simulink model "vipldws"  (R2017b)
settings: Solver=FixedStepDiscrete  StartTime=0.0  StopTime=inf  RelTol=1e-3  EnableMultiTasking=on
model workspace (MATLAB code in the model file):
  | % Image size
  | imgSize = [240 360];
  | 
  | % Number of rows and columns in the image region to process.
  | numRows = floor(imgSize(1)/2);
  | numCols = imgSize(2);
  | 
  | % To handle different video sizes other than [240 360], scaling the Hough
  | % transform rho values by the below factor is required.
  | factor = sqrt(sum(imgSize.^2)) / sqrt(sum([240 360].^2));
  | 
  | %% parameters for the second lane
  | %approximately 35:45 (0-based index: 414:424)
  | startIdxRho_R = floor(factor * 414);
  | NumRhos_R = floor(factor * 11);
  | 
  | %approximately -90:-70 degrees (0-based index: 0:20)
  | startIdxTheta_R = 0;
  | NumThetas_R = 21;
  | neighborhood_R =  [min(7,NumRhos_R), min(7,NumThetas_R)];
  | 
  | %approximately 379:415 (0-based index: 0:35)
  | startIdxRho_L = floor(factor * 379);
  | NumRhos_L = floor(factor * 36);
  | 
  | %approximately 55:85 degrees (0-based index: 145: 175)
  | startIdxTheta_L = 145;
  | NumThetas_L = 21;
  | neighborhood_L =  [min(7,NumRhos_L), min(7,NumThetas_L)];
  | 
  | % Maximum number of lanes to find in the current frame.
  | expLaneNum = 2;
  | 
  | % Maximum number of lanes to store in the tracking repository.
  | maxLaneNum = 20;
  | 
  | % Angular resolution of Hough transform, i.e., the width of a theta bin is
  | % pi/angleNum.
  | angleNum = 180;
  | 
  | % Maximum allowable change of lane distance metric between two frames.
  | trackThreshold = 75;
  | 
  | % Minimum number of frames a lane must be detected to become a valid lane.
  | frameFound = 5;
  | 
  | % Maximum number of frames a lane can be missed without marking it invalid.
  | frameLost = 20;
  | 
  | % Size of the neighborhood around the maxima over which the Hough
  | % transforms values are suppressed. (Used in Find Local Maxima block)
  | neighborhood = [301, 81];
  | 
  | % Distance threshold for lane crossing warning; valid range is (0, 0.5).
  | thrWarn = 0.4;
  | 
  | % Weight (tweaking factor) of the angular difference for calculating the
  | % distance metric between two lanes. It is typically chosen to be close
  | % to the input image rows.
  | distanceMetricWeight = 200;
  | 
  | % Audio track used for lane cross warning.
  | load viprumbling.mat;
undefined symbols (not defined in the file or in its folder): gray, High, num_targets, Rec, SDTV, slselsubs
libraries: simulink x17, visiontextngfix x6, visiontransforms x4, dspmtrx3 x3, visionconversions x3, visionstatistics x3, dspindex x2, dspswit3 x2, dspstat3 x2, simulink_need_slupdate x2, dspsigops x1, vipmisc x1
(part 2 of 2)

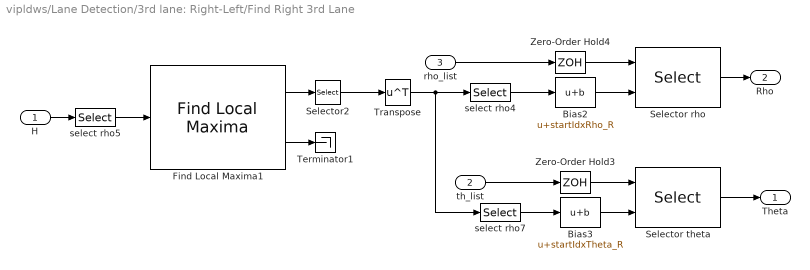
== system vipldws/Lane Detection/3rd lane: Right-Left/Find Right 3rd Lane ==
  H : Inport
  th_list : Inport  Port=2
  rho_list : Inport  Port=3
  Bias2 : Bias  Bias=startIdxRho_R
  Bias3 : Bias  Bias=startIdxTheta_R
  Find Local Maxima1 : visionstatistics/Find Local Maxima  num_peaks=1  nhood_size=neighborhood_R  src_thresh=Obsolete9b  src_thresh_inuse=Specify via dialog  threshold=1  inputIsHough=on  dt_peak=uint16  isOutVarDim=off  dt_count=uint16
      settings: SourceProductName=Computer Vision System Toolbox  SourceProductBaseCode=VP
  Selector rho : Selector  NumberOfDimensions=2  InputPortWidth=3  IndexOptions=Select all,Index vector (port)  Indices=1,2  OutputSizes=1,1
  Selector theta : Selector  NumberOfDimensions=2  InputPortWidth=3  IndexOptions=Select all,Index vector (port)  Indices=1,2  OutputSizes=1,1
  Selector2 : Selector  NumberOfDimensions=2  InputPortWidth=3  IndexOptions=Select all,Index vector (dialog)  Indices=,[2 1]  OutputSizes=1,1
  Terminator1 : Terminator
  Transpose : Math  Operator=transpose  SaturateOnIntegerOverflow=on
  Zero-Order Hold3 : ZeroOrderHold  SampleTime=-1
  Zero-Order Hold4 : ZeroOrderHold  SampleTime=-1
  select rho4 : Selector  NumberOfDimensions=2  InputPortWidth=3  IndexOptions=Index vector (dialog),Select all  Indices=1,-1  OutputSizes=1
  select rho5 : Selector  NumberOfDimensions=2  IndexMode=Zero-based  InputPortWidth=3  IndexOptions=Index vector (dialog),Index vector (dialog)  Indices=startIdxRho_R:(startIdxRho_R+NumRhos_R-1),startIdxTheta_R:(startIdxTheta_R+NumThetas_R-1)  OutputSizes=1
  select rho7 : Selector  NumberOfDimensions=2  InputPortWidth=3  IndexOptions=Index vector (dialog),Select all  Indices=2,-1  OutputSizes=1
  Theta : Outport
  Rho : Outport  Port=2
  wires:
  select rho4/1 -> Bias2/1
  Selector theta/1 -> Theta/1
  H/1 -> select rho5/1
  Find Local Maxima1/2 -> Terminator1/1
  Selector rho/1 -> Rho/1
  Bias3/1 -> Selector theta/2
  Bias2/1 -> Selector rho/2
  select rho7/1 -> Bias3/1
  select rho5/1 -> Find Local Maxima1/1
  rho_list/1 -> Zero-Order Hold4/1
  Zero-Order Hold4/1 -> Selector rho/1
  th_list/1 -> Zero-Order Hold3/1
  Zero-Order Hold3/1 -> Selector theta/1
  Selector2/1 -> Transpose/1
  Find Local Maxima1/1 -> Selector2/1
  Transpose/1 -> select rho7/1, select rho4/1

== system vipldws/Lane Detection/Peak detection/Enable signal generator ==
  Num : Inport
  Assignment : Assignment  NumberOfDimensions=2  IndexOptions=Assign all,Index vector (port)  Indices=-1,1  OutputSizes=1,1
  Constant : Constant  Value=zeros(1, expLaneNum)  VectorParams1D=off  OutDataTypeStr=boolean
  Constant1 : Constant  VectorParams1D=off  OutDataTypeStr=boolean
  For Iterator : ForIterator  ResetStates=reset  IterationSource=external
  Enable : Outport
  wires:
  For Iterator/1 -> Assignment/3
  Constant1/1 -> Assignment/2
  Assignment/1 -> Enable/1
  Constant/1 -> Assignment/1
  Num/1 -> For Iterator/1

== system vipldws/Lane Tracking/Matching/Calculate the distances between the lines found in the current frame and those in the repository ==
  Count : Inport
  Rep_ref : Inport  Port=2
  Line : Inport  Port=3
  Enable : Inport  Port=4
  For Iterator : ForIterator  ResetStates=reset  IterationLimit=maxLaneNum
  "Select a line from the repository; if it is valid (Count > 0), Calculate its distance to the input lines." : Subsystem
  Selector1 : Selector  NumberOfDimensions=2  InputPortWidth=3  IndexOptions=Select all,Index vector (port)  Indices=-1,-1  OutputSizes=1
  Dis : Outport
  wires:
  Enable/1 -> "Select a line from the repository; if it is valid (Count > 0), Calculate its distance to the input lines."/4(Enable)
  For Iterator/1 -> Selector1/2, "Select a line from the repository; if it is valid (Count > 0), Calculate its distance to the input lines."/1(Idx)
  "Select a line from the repository; if it is valid (Count > 0), Calculate its distance to the input lines."/1(Dis) -> Dis/1
  Rep_ref/1 -> "Select a line from the repository; if it is valid (Count > 0), Calculate its distance to the input lines."/2(Rep_ref)
  Line/1 -> "Select a line from the repository; if it is valid (Count > 0), Calculate its distance to the input lines."/3(Line)
  Count/1 -> Selector1/1
  Selector1/1 -> "Select a line from the repository; if it is valid (Count > 0), Calculate its distance to the input lines."/Enable

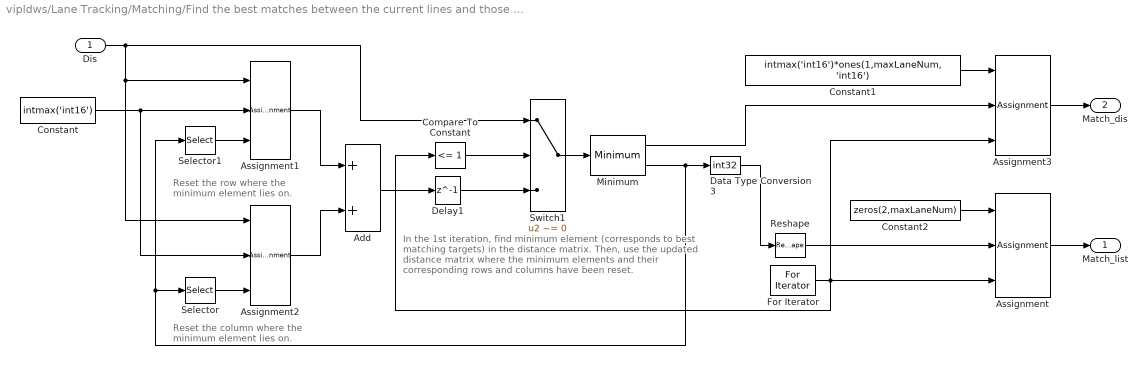
== system vipldws/Lane Tracking/Matching/Find the best matches between the current lines and those in the repository ==
  note: In the 1st iteration, find minimum element (corresponds to
      | best matching targets) in the distance matrix. Then, use the
      | updated distance matrix where the minimum elements and
      | their  corresponding rows and columns have been reset.
  note: Reset the column where the
      | minimum element lies on.
  note: Reset the row where the
      | minimum element lies on.
  Dis : Inport
  Add : Sum
  Assignment : Assignment  NumberOfDimensions=2  IndexOptions=Assign all,Index vector (port)  Indices=-1,-1  OutputSizes=1,1
  Assignment1 : Assignment  NumberOfDimensions=2  IndexOptions=Index vector (port),Assign all  Indices=1,-1  OutputSizes=1,1
  Assignment2 : Assignment  NumberOfDimensions=2  IndexOptions=Assign all,Index vector (port)  Indices=-1,-1  OutputSizes=1,1
  Assignment3 : Assignment  NumberOfDimensions=2  IndexOptions=Assign all,Index vector (port)  Indices=-1,-1  OutputSizes=1,1
  Compare To Constant : simulink/Logic and Bit Operations/Compare To Constant  relop=<=  const=1  OutDataTypeStr=boolean  ZeroCross=off
  Constant : Constant  Value=intmax('int16')  VectorParams1D=off  OutDataTypeStr=Inherit: Inherit via back propagation
  Constant1 : Constant  Value=intmax('int16')*ones(1,maxLaneNum, 'int16')  VectorParams1D=off  OutDataTypeStr=Inherit: Inherit via back propagation
  Constant2 : Constant  Value=zeros(2,maxLaneNum)  VectorParams1D=off  OutDataTypeStr=Inherit: Inherit via back propagation
  Data Type Conversion3 : DataTypeConversion  OutDataTypeStr=int32  SaturateOnIntegerOverflow=on  RndMeth=Zero
  Delay1 : Delay  DelayLength=1  InitialCondition=0  UseCircularBuffer=on
  For Iterator : ForIterator  IterationLimit=expLaneNum
  Minimum : dspstat3/Minimum  operation=minimum  fcn=Value and Index  indexBase=One  operateOver=Entire input  Dimension=1  InputProcessing=Columns as channels (frame based)  reset=None  roiEnable=off  roiType=Rectangles  roiPortion=Entire ROI  roiOutput=Individual statistics for each ROI  roiFlag=off  roundingMode=Floor  overflowMode=off
      settings: SourceProductName=DSP System Toolbox  SourceProductBaseCode=DS
  Reshape : Reshape  OutputDimensionality=Column vector (2-D)
  Selector : Selector  InputPortWidth=2  IndexOptions=Index vector (dialog)  Indices=[2]  OutputSizes=1
  Selector1 : Selector  InputPortWidth=2  IndexOptions=Index vector (dialog)  Indices=[1]  OutputSizes=1
  Switch1 : Switch  Criteria=u2 ~= 0
  Match_list : Outport
  Match_dis : Outport  Port=2
  wires:
  Constant2/1 -> Assignment/1
  Constant1/1 -> Assignment3/1
  Data Type Conversion3/1 -> Reshape/1
  Compare To Constant/1 -> Switch1/2
  For Iterator/1 -> Compare To Constant/1, Assignment/3, Assignment3/3
  Switch1/1 -> Minimum/1
  Dis/1 -> Assignment2/1, Assignment1/1, Switch1/1
  Delay1/1 -> Switch1/3
  Assignment/1 -> Match_list/1
  Selector/1 -> Assignment2/3
  Selector1/1 -> Assignment1/3
  Assignment1/1 -> Add/1
  Assignment2/1 -> Add/2
  Add/1 -> Delay1/1
  Assignment3/1 -> Match_dis/1
  Minimum/2 -> Data Type Conversion3/1, Selector/1, Selector1/1
  Minimum/1 -> Assignment3/2
  Constant/1 -> Assignment1/2, Assignment2/2
  Reshape/1 -> Assignment/2

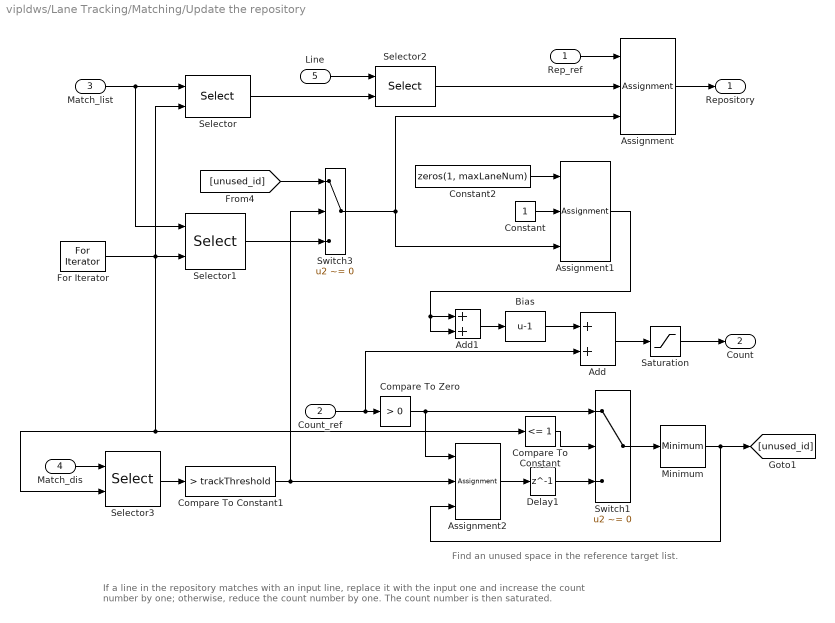
== system vipldws/Lane Tracking/Matching/Update the repository ==
  note: Find an unused space in the reference target list.
  note: If a line in the repository matches with an input line, replace it with the input one and increase the count number by one;
      | otherwise, reduce the count number by one. The count number is then saturated.
  Rep_ref : Inport
  Count_ref : Inport  Port=2
  Match_list : Inport  Port=3
  Match_dis : Inport  Port=4
  Line : Inport  Port=5
  Add : Sum  InputSameDT=on
  Add1 : Sum  OutDataTypeStr=int32  InputSameDT=on
  Assignment : Assignment  NumberOfDimensions=2  IndexOptions=Assign all,Starting index (port)  Indices=-1,-1  OutputSizes=1,1
  Assignment1 : Assignment  NumberOfDimensions=2  IndexOptions=Assign all,Index vector (port)  Indices=-1,-1  OutputSizes=slselsubs([1, num_targets],1),slselsubs([1, num_targets],2)
  Assignment2 : Assignment  IndexOptions=Index vector (port)  Indices=-1  OutputSizes=[1, num_targets]
  Bias : Bias  Bias=-1
  Compare To Constant : simulink/Logic and Bit Operations/Compare To Constant  relop=<=  const=1  OutDataTypeStr=boolean  ZeroCross=off
  Compare To Constant1 : simulink/Logic and Bit Operations/Compare To Constant  relop=>  const=trackThreshold  OutDataTypeStr=boolean  ZeroCross=off
  Compare To Zero : simulink/Logic and Bit Operations/Compare To Zero  relop=>  OutDataTypeStr=boolean  ZeroCross=off
  Constant : Constant  VectorParams1D=off  OutDataTypeStr=Inherit: Inherit via back propagation
  Constant2 : Constant  Value=zeros(1, maxLaneNum)  VectorParams1D=off  OutDataTypeStr=int32
  Delay1 : Delay  DelayLength=1  InitialCondition=0  UseCircularBuffer=on
  For Iterator : ForIterator  ResetStates=reset  IterationLimit=expLaneNum
  Minimum : dspstat3/Minimum  operation=minimum  fcn=Index  indexBase=One  operateOver=Each row  Dimension=1  InputProcessing=Columns as channels (frame based)  reset=None  roiEnable=off  roiType=Rectangles  roiPortion=Entire ROI  roiOutput=Individual statistics for each ROI  roiFlag=off  roundingMode=Floor  overflowMode=off
      settings: SourceProductName=DSP System Toolbox  SourceProductBaseCode=DS
  Saturation : Saturate  UpperLimit=frameFound+frameLost  LowerLimit=0
  Selector : Selector  NumberOfDimensions=2  InputPortWidth=3  IndexOptions=Index vector (dialog),Index vector (port)  Indices=[2],[1]  OutputSizes=1
  Selector1 : Selector  NumberOfDimensions=2  InputPortWidth=3  IndexOptions=Index vector (dialog),Index vector (port)  Indices=[1],[2]  OutputSizes=1
  Selector2 : Selector  NumberOfDimensions=2  InputPortWidth=3  IndexOptions=Select all,Index vector (port)  Indices=-1,1  OutputSizes=1
  Selector3 : Selector  NumberOfDimensions=2  InputPortWidth=3  IndexOptions=Select all,Index vector (port)  Indices=-1,-1  OutputSizes=1
  Switch1 : Switch  Criteria=u2 ~= 0
  Switch3 : Switch  Criteria=u2 ~= 0
  Repository : Outport
  Count : Outport  Port=2
  wires:
  Constant2/1 -> Assignment1/1
  Constant/1 -> Assignment1/2
  Switch3/1 -> Assignment1/3, Assignment/3
  Selector1/1 -> Switch3/3
  Selector/1 -> Selector2/2
  [unused_id] -> Switch3/1
  Compare To Constant1/1 -> Switch3/2, Assignment2/2
  Delay1/1 -> Switch1/3
  Count_ref/1 -> Add/2, Compare To Zero/1
  Switch1/1 -> Minimum/1
  Minimum/1 -> [unused_id], Assignment2/3
  Assignment2/1 -> Delay1/1
  Match_dis/1 -> Selector3/1
  Assignment1/1 -> Add1/1, Add1/2
  Assignment/1 -> Repository/1
  Line/1 -> Selector2/1
  Match_list/1 -> Selector/1, Selector1/1
  Compare To Constant/1 -> Switch1/2
  For Iterator/1 -> Selector3/2, Compare To Constant/1, Selector/2, Selector1/2
  Selector2/1 -> Assignment/2
  Add1/1 -> Bias/1
  Bias/1 -> Add/1
  Add/1 -> Saturation/1
  Compare To Zero/1 -> Switch1/1, Assignment2/1
  Rep_ref/1 -> Assignment/1
  Selector3/1 -> Compare To Constant1/1
  Saturation/1 -> Count/1

== system vipldws/Output/Subsystem/Draw  Polygon ==
  inPts : Inport
  RGB : Inport  Port=2
  Enable : EnablePort  PropagateVarSize=During execution
  DrawShapes : visiontextngfix/Draw Shapes  shape=Polygons  fill=on  lineWidth=1  fillClrSource=Specify via dialog  display=User-specified value  intensity=200  color=[0 1 1]  opacity=0.2  viewport=Entire image  antialiasing=off  inType=Obsolete  imagePorts=One multidimensional signal  prodOutputMode=Binary point scaling  prodOutputWordLength=32  prodOutputFracLength=14  memoryMode=Specify word length  memoryWordLength=16  memoryFracLength=14  roundingMode=Floor  overflowMode=off
      settings: SourceProductName=Computer Vision System Toolbox
  Line to Polygon Coordinates : Subsystem
  Selector2 : Selector  NumberOfDimensions=2  InputPortWidth=3  IndexOptions=Index vector (dialog),Select all  Indices=[2 1 4 3 6 5 8 7 10 9 12 11],1  OutputSizes=1,1
  Transpose1 : Math  Operator=transpose  SaturateOnIntegerOverflow=on
  RGBout : Outport
  wires:
  RGB/1 -> DrawShapes/1
  DrawShapes/1 -> RGBout/1
  inPts/1 -> Line to Polygon Coordinates/1(Pts_line)
  Selector2/1 -> Transpose1/1
  Line to Polygon Coordinates/1(Pts_polygon) -> Selector2/1
  Transpose1/1 -> DrawShapes/2

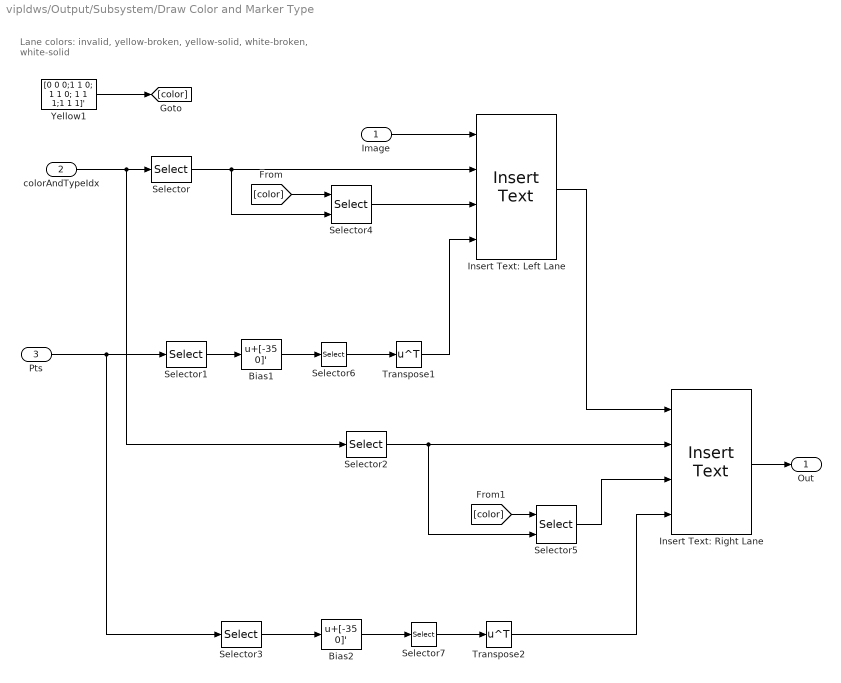
== system vipldws/Output/Subsystem/Draw Color and Marker Type ==
  note: Lane colors:
      | invalid, yellow-broken, yellow-solid, white-broken, white-solid
  Image : Inport
  colorAndTypeIdx : Inport  Port=2
  Pts : Inport  Port=3
  Bias1 : Bias  Bias=[-35 0]'
  Bias2 : Bias  Bias=[-35 0]'
  Insert Text: Left Lane : visiontextngfix/Insert Text  inputType=Obsolete  theText={'',sprintf('Yellow\nBroken'),sprintf('Yellow\nSolid'),sprintf('White\nBroken'),sprintf('White\nSolid')}  getTextLocFrom=Input port  textLoc=[170 2]  getTextColorFrom=Input port  textColor=[1 1 1]  getTextIntensityFrom=Specify via dialog  textIntensity=0  getTextOpacityFrom=Specify via dialog  textOpacity=1  dummyVar2=0  dummyVar3=0  dummyVar4=0  imagePorts=One multidimensional signal  isInputTransposed=off  fontFace=LucidaTypewriterBold  dummyVar1=0  blockFontSize=14  antiAliased=on
      settings: SourceProductName=Computer Vision System Toolbox  SourceProductBaseCode=VP
  Insert Text: Right Lane : visiontextngfix/Insert Text  inputType=Obsolete  theText={'',sprintf('Yellow\nBroken'),sprintf('Yellow\nSolid'),sprintf('White\nBroken'),sprintf('White\nSolid')}  getTextLocFrom=Input port  textLoc=[170 2]  getTextColorFrom=Input port  textColor=[1 1 1]  getTextIntensityFrom=Specify via dialog  textIntensity=0  getTextOpacityFrom=Specify via dialog  textOpacity=1  dummyVar2=0  dummyVar3=0  dummyVar4=0  imagePorts=One multidimensional signal  isInputTransposed=off  fontFace=LucidaTypewriterBold  dummyVar1=0  blockFontSize=14  antiAliased=on
      settings: SourceProductName=Computer Vision System Toolbox  SourceProductBaseCode=VP
  Selector : Selector  IndexMode=Zero-based  InputPortWidth=2  IndexOptions=Index vector (dialog)  Indices=0  OutputSizes=1
  Selector1 : Selector  NumberOfDimensions=2  IndexMode=Zero-based  InputPortWidth=2  IndexOptions=Index vector (dialog),Index vector (dialog)  Indices=[0 1],0  OutputSizes=1,1
  Selector2 : Selector  IndexMode=Zero-based  InputPortWidth=2  IndexOptions=Index vector (dialog)  Indices=1  OutputSizes=1
  Selector3 : Selector  NumberOfDimensions=2  IndexMode=Zero-based  InputPortWidth=2  IndexOptions=Index vector (dialog),Index vector (dialog)  Indices=0:1,1  OutputSizes=1,1
  Selector4 : Selector  NumberOfDimensions=2  InputPortWidth=3  IndexOptions=Select all,Index vector (port)  Indices=[1 3],1  OutputSizes=1,1
  Selector5 : Selector  NumberOfDimensions=2  InputPortWidth=3  IndexOptions=Select all,Index vector (port)  Indices=[1 3],1  OutputSizes=1,1
  Selector6 : Selector  NumberOfDimensions=2  InputPortWidth=3  IndexOptions=Index vector (dialog),Select all  Indices=[2 1],[2 1]  OutputSizes=1,1
  Selector7 : Selector  NumberOfDimensions=2  InputPortWidth=3  IndexOptions=Index vector (dialog),Select all  Indices=[2 1],1  OutputSizes=1,1
  Transpose1 : Math  Operator=transpose  SaturateOnIntegerOverflow=on
  Transpose2 : Math  Operator=transpose  SaturateOnIntegerOverflow=on
  Yellow1 : Constant  Value="[0 0  0;1 1 0; 1 1 0; 1 1 1;1 1 1]'"  VectorParams1D=off  OutDataTypeStr=single
  Out : Outport
  wires:
  Selector4/1 -> Insert Text: Left Lane/3
  Selector/1 -> Insert Text: Left Lane/2, Selector4/2
  Selector1/1 -> Bias1/1
  Image/1 -> Insert Text: Left Lane/1
  colorAndTypeIdx/1 -> Selector/1, Selector2/1
  Insert Text: Left Lane/1 -> Insert Text: Right Lane/1
  Pts/1 -> Selector1/1, Selector3/1
  Selector5/1 -> Insert Text: Right Lane/3
  Selector3/1 -> Bias2/1
  Insert Text: Right Lane/1 -> Out/1
  [color] -> Selector4/1
  [color] -> Selector5/1
  Yellow1/1 -> [color]
  Selector6/1 -> Transpose1/1
  Selector7/1 -> Transpose2/1
  Bias2/1 -> Selector7/1
  Bias1/1 -> Selector6/1
  Transpose1/1 -> Insert Text: Left Lane/4
  Transpose2/1 -> Insert Text: Right Lane/4
  Selector2/1 -> Selector5/2, Insert Text: Right Lane/2

== system vipldws/Lane Tracking/Matching/Calculate the distances between the lines found in the current frame and those in the repository/Select a line from the repository; if it is valid (Count > 0), Calculate its distance to the input lines. ==
  Idx : Inport
  Rep_ref : Inport  Port=2
  Line : Inport  Port=3
  Enable : Inport  Port=4
  EnablePort : EnablePort  StatesWhenEnabling=reset  PropagateVarSize=During execution
  Assignment : Assignment  NumberOfDimensions=2  IndexOptions=Index vector (port),Assign all  Indices=-1,-1  OutputSizes=1,1
  Calculate the distances between the chosen line in the repository and all input lines. : Subsystem  TreatAsAtomicUnit=on
  Constant2 : Constant  Value=intmax('int16') * ones(maxLaneNum,'int16')  VectorParams1D=off  OutDataTypeStr=int32
  Selector1 : Selector  NumberOfDimensions=2  InputPortWidth=3  IndexOptions=Index vector (port),Select all  Indices=-1,-1  OutputSizes=1
  Selector2 : Selector  NumberOfDimensions=2  InputPortWidth=3  IndexOptions=Select all,Index vector (port)  Indices=-1,-1  OutputSizes=1
  Dis : Outport
  wires:
  Rep_ref/1 -> Selector2/1
  Enable/1 -> Calculate the distances between the chosen line in the repository and all input lines./4(Enable)
  Selector2/1 -> Calculate the distances between the chosen line in the repository and all input lines./2(Rep_ref)
  Line/1 -> Calculate the distances between the chosen line in the repository and all input lines./3(Line)
  Selector1/1 -> Calculate the distances between the chosen line in the repository and all input lines./1(Dis)
  Idx/1 -> Selector2/2, Assignment/3, Selector1/2
  Assignment/1 -> Dis/1
  Calculate the distances between the chosen line in the repository and all input lines./1(Dis_out) -> Assignment/2
  Constant2/1 -> Selector1/1, Assignment/1

== system vipldws/Output/Subsystem/Draw  Polygon/Line to Polygon Coordinates ==
  note: r1   R1
      | c1   C1
      | r2   R2
      | c2   C2
  note: r1
      | c1
  note: R1
      | C1
  note: (r1,c1)
      |                        /
      |                    /
      |               /
      |          /
      | (r2,c2)
  note: (R1,C1)
      |  \
      |        \
      |            \
      |                  \
      |                        (R2,C2)
  note: R2
      | C2
  note: r1
      | c1
      | ----
      | r2
      | c2
      | ----
      | r2     or   239
      | c2     or    0
      | ------
      | R2    or    239
      | C2    or    359
      | -----
      | R2
      | C2
      | -----
      | R1
      | C1
  note: r2
      | c2
  note: r2
      | c2
  note: r2     or   239
      | c2     or    0
  note: R2
      | C2
  note: R2    or    239
      | C2    or    359
  Pts_line : Inport
  DSP Constant : Constant  Value=[239 0]'  VectorParams1D=off  OutDataTypeStr=int32  SampleTime=1/30
  DSP Constant2 : Constant  Value=[239 359]'  VectorParams1D=off  OutDataTypeStr=int32  SampleTime=1/30
  Matrix Concatenation6 : Concatenate  NumInputs=6  Mode=Multidimensional array
  Selector : Selector  NumberOfDimensions=2  InputPortWidth=3  IndexOptions=Index vector (dialog),Index vector (dialog)  Indices=3:4,2  OutputSizes=1
  Selector1 : Selector  NumberOfDimensions=2  InputPortWidth=3  IndexOptions=Index vector (dialog),Index vector (dialog)  Indices=1:2,1  OutputSizes=1
  Selector2 : Selector  NumberOfDimensions=2  InputPortWidth=3  IndexOptions=Index vector (dialog),Index vector (dialog)  Indices=1:2,2  OutputSizes=1
  Selector3 : Selector  InputPortWidth=2  IndexOptions=Index vector (dialog)  Indices=1  OutputSizes=1
  Selector4 : Selector  NumberOfDimensions=2  InputPortWidth=3  IndexOptions=Index vector (dialog),Index vector (dialog)  Indices=3:4,1  OutputSizes=1
  Selector5 : Selector  InputPortWidth=2  IndexOptions=Index vector (dialog)  Indices=1  OutputSizes=1
  Switch : Switch  Threshold=239
  Switch1 : Switch  Threshold=239
  Pts_polygon : Outport
  wires:
  Selector1/1 -> Matrix Concatenation6/1
  Selector/1 -> Switch1/1, Selector5/1, Matrix Concatenation6/5
  Matrix Concatenation6/1 -> Pts_polygon/1
  Selector3/1 -> Switch/2  "r2"
  Selector4/1 -> Switch/1, Selector3/1, Matrix Concatenation6/2
  DSP Constant/1 -> Switch/3
  Selector5/1 -> Switch1/2  "R2"
  DSP Constant2/1 -> Switch1/3
  Selector2/1 -> Matrix Concatenation6/6
  Switch/1 -> Matrix Concatenation6/3
  Switch1/1 -> Matrix Concatenation6/4
  Pts_line/1 -> Selector1/1, Selector4/1, Selector/1, Selector2/1

== system vipldws/Lane Tracking/Matching/Calculate the distances between the lines found in the current frame and those in the repository/Select a line from the repository; if it is valid (Count > 0), Calculate its distance to the input lines./Calculate the distances between the chosen line in the repository and all input lines. ==
  note: Calculate the distance between the chosen line in the repository and every input line.
  Dis : Inport
  Rep_ref : Inport  Port=2
  Line : Inport  Port=3
  Enable : Inport  Port=4
  Assignment : Assignment  IndexOptions=Index vector (port)  Indices=1  OutputSizes=[1 1]
  Constant : Constant  Value=intmax('int16')  VectorParams1D=off  OutDataTypeStr=int32
  Difference between two lines : Subsystem
  For Iterator : ForIterator  ResetStates=reset  IterationLimit=expLaneNum
  Selector1 : Selector  NumberOfDimensions=2  InputPortWidth=3  IndexOptions=Select all,Index vector (port)  Indices=-1,-1  OutputSizes=1
  Selector2 : Selector  NumberOfDimensions=2  InputPortWidth=3  IndexOptions=Select all,Index vector (port)  Indices=-1,-1  OutputSizes=1
  Switch1 : Switch  Criteria=u2 ~= 0
  Dis_out : Outport
  wires:
  Selector1/1 -> Difference between two lines/2(Line_2)
  Constant/1 -> Switch1/3
  Difference between two lines/1(Dis) -> Switch1/1
  Selector2/1 -> Switch1/2, Difference between two lines/Enable
  Enable/1 -> Selector2/1
  Line/1 -> Selector1/1
  For Iterator/1 -> Selector1/2, Selector2/2, Assignment/3
  Rep_ref/1 -> Difference between two lines/1(Line_1)
  Dis/1 -> Assignment/1
  Assignment/1 -> Dis_out/1
  Switch1/1 -> Assignment/2

== system vipldws/Lane Tracking/Matching/Calculate the distances between the lines found in the current frame and those in the repository/Select a line from the repository; if it is valid (Count > 0), Calculate its distance to the input lines./Calculate the distances between the chosen line in the repository and all input lines./Difference between two lines ==
  note: Distance between two lines equals to
      | abs( Rho1 - Rho2) + abs( Theta1 - Theta2) * estImageSize,
      | where estImageSize is the estimated size of the image.
  Line_1 : Inport
  Line_2 : Inport  Port=2
  Enable : EnablePort  PropagateVarSize=During execution
  Abs : Abs
  Abs1 : Abs
  Add1 : Sum  Inputs=+-  OutDataTypeStr=int32
  Add7 : Sum  OutDataTypeStr=Inherit: Same as first input
  Add8 : Sum  Inputs=+-
  Constant : Constant
  Constant1 : Constant  Value=2
  Gain : Gain  Gain=distanceMetricWeight  OutDataTypeStr=Inherit: Inherit via back propagation
  Rho_1 : Selector  InputPortWidth=2  IndexOptions=Index vector (dialog)  Indices=1  OutputSizes=1
  Rho_2 : Selector  InputPortWidth=2  IndexOptions=Index vector (port)  Indices=1  OutputSizes=1
  Theta_1 : Selector  InputPortWidth=2  IndexOptions=Index vector (dialog)  Indices=2  OutputSizes=1
  Theta_2 : Selector  InputPortWidth=2  IndexOptions=Index vector (port)  Indices=2  OutputSizes=1
  Dis : Outport
  wires:
  Line_1/1 -> Rho_1/1, Theta_1/1
  Line_2/1 -> Rho_2/1, Theta_2/1
  Theta_1/1 -> Add8/1
  Theta_2/1 -> Add8/2
  Add8/1 -> Abs/1
  Add7/1 -> Dis/1
  Abs/1 -> Gain/1
  Add1/1 -> Abs1/1
  Rho_1/1 -> Add1/1
  Rho_2/1 -> Add1/2
  Abs1/1 -> Add7/1
  Gain/1 -> Add7/2
  Constant/1 -> Rho_2/2
  Constant1/1 -> Theta_2/2

== matlab function vipldws/Output/Exclude 3rd Lane ==
  data: in3rdLane input; out3rdLane output; Show3rdLane input; mainTwoLanes input; twoLanesFlag input; RefImg input
function out3rdLane =Exclude3rdLane(in3rdLane, Show3rdLane, mainTwoLanes, twoLanesFlag, RefImg)  

% Exclude third (left or right lane) if it is very close to the other lane 
% already detected and tracked by Kalman filter.

[rH cW] = size(RefImg(:,:,1));
out3rdLane = in3rdLane;  

if (Show3rdLane && twoLanesFlag)
    R1C1R2C2 = in3rdLane;
    R1 = R1C1R2C2(1)+int32(1); 
    C1 = R1C1R2C2(2)+int32(1); 
    R2 = R1C1R2C2(3)+int32(1);  
    C2 = R1C1R2C2(4)+int32(1);  
    % make sure R1 is the min(R1,R2)
    if R1>R2
        TMP=R2;
        R2=R1;
        R1=TMP;

        TMP=C2;
        C2=C1;
        C1=TMP;   
    end
    
  for lineIdx =1:2  
    
    r1c1r2c2 = mainTwoLanes(:,lineIdx);
    r1 = r1c1r2c2(1)+int32(1);  
    c1 = r1c1r2c2(2)+int32(1);  
    r2 = r1c1r2c2(3)+int32(1);  
    c2 = r1c1r2c2(4)+int32(1); 

    % make sure r1 is the min(r1,r2)
    if r1>r2
        tmp=r2;
        r2=r1;
        r1=tmp;

        tmp=c2;
        c2=c1;
        c1=tmp;   
    end
    
    pointNotLine = (r1==r2) && (c1==c2);
    
    % find if line is within image: (r1,c1)  and (r2,c2) must be within image
    if ((r1>0 && r1 <= rH) && (c1>0 && c1 <= cW) && ...
        (r2>0 && r2 <= rH) && (c2>0 && c2 <= cW)) && ~pointNotLine
        %line_within_image = true;
        if (abs(r1-R1)+ abs(c1-C1) + abs(r2-R2) +abs(c2-C2))< int32(20)
            out3rdLane = int32([-1000 -1000 -1000 -1000]');
        end            
    else
       % line outside image
       % go to nextLine
    end    
  end    
else
   out3rdLane = in3rdLane;  
end

== matlab function vipldws/Departure Warning/Departure detection/subsystem/Combine Left Right Departure ==
  data: curMsg input; prevMsg input int8; outMsg output; numNormalDrivenFrames input
function outMsg=CombineLeftRightDeparture(curMsg, prevMsg, numNormalDrivenFrames)  

% It combines left-right departure to left departure
%         and right-left departure to right departure
% It utilizes the fact that there must be at least 4 frames of normal driving 
% between a left departure warning and a right departure warning

%RIGHT_DEP=0; NORMAL=1; LEFT_DEP=2
NORMAL = int8(1);

if curMsg == NORMAL
    outMsg = NORMAL;
else % curMsg == RIGHT_DEP  || curMsg == LEFT_DEP
    if (numNormalDrivenFrames < int32(4))
        % use the previous message
        outMsg = prevMsg;        
    else
        outMsg = curMsg;
    end        
end

== matlab function vipldws/Departure Warning/Departure detection/DetectColorAndType1 ==
  data: twoLines_0b input; colorAndTypeIdx output; YCbCr input
function colorAndTypeIdx =DetectColorAndType(twoLines_0b, YCbCr)  

% Detects if the lane detected is Yellow/White and Solid/Broken
% twoLines_0b =  coordinate points of lines (0 based)

% Here, for a line with start point (r1,c1) and end point (r2,c2),
% we form a ROI with points: 
% (r1,c1-HALF_OFFSET) (r1,c1+HALF_OFFSET) 
% (r2,c2-HALF_OFFSET) (r2,c2+HALF_OFFSET) 
% We search for yellow/white color within this ROI 

INVALID_COLOR = int8(0);
WHITE_COLOR   = int8(1);
YELLOW_COLOR  = int8(2); 

INVALID_MARKING = int8(0);
BROKEN_MARKING  = int8(1); 
SOLID_MARKING   = int8(2);

INVALID_COLOR_OR_TYPE = int8(0);% color=yellow/white; type=broken or solid
YELLOW_BROKEN  = int8(1); 
YELLOW_SOLID   = int8(2); 
WHITE_BROKEN   = int8(3); 
WHITE_SOLID    = int8(4); 

lineColorIdx    = int8([0 0]);
solidBrokenIdx  = int8([0 0]);
colorAndTypeIdx = int8([0 0]);
HALF_OFFSET =  int32(10);

zeroI32 = int32(0);
oneI32  = int32(1);
twoI32  = int32(2);

rH = int32(size(YCbCr(:,:,1),1));
cW = int32(size(YCbCr(:,:,1),2));

tmpInImage_Y  = YCbCr(:,:,1);
tmpInImage_Cb = YCbCr(:,:,2);

leftC  = int32(zeros(rH,1));
rightC = int32(zeros(rH,1));
Rs     = int32(zeros(rH,1));

%twoLines_1b = twoLines_0b+int32(1);
twoLines_1b = twoLines_0b;
for i=oneI32:int32(length(twoLines_1b(:)))
    twoLines_1b(i) = twoLines_1b(i) + oneI32;
end

for lineIdx =oneI32:twoI32%1:2
    %% one line
    r1c1r2c2 = twoLines_1b(:,lineIdx);
    r1 = r1c1r2c2(1); 
    c1 = r1c1r2c2(2); 
    r2 = r1c1r2c2(3); 
    c2 = r1c1r2c2(4); 

    % make sure r1 is the min (r1,r2)
    if r1>r2
        tmp=r2;
        r2=r1;
        r1=tmp;

        tmp=c2;
        c2=c1;
        c1=tmp;   
    end

    pointNotLine = (r1==r2) && (c1==c2);
    
    % find if line is within image: (r1,c1)  and (r2,c2) must be within image
    if ((r1>zeroI32 && r1 <= rH) && (c1>zeroI32 && c1 <= cW) && ...
        (r2>zeroI32 && r2 <= rH) && (c2>zeroI32 && c2 <= cW)) && ~pointNotLine
        line_within_image = logical(true);
    else
        line_within_image = logical(false);
    end

    if (line_within_image)
        len = r2-r1+oneI32;
        i=oneI32;
        % Rs(1:len)=r1:r2
        for p=r1:r2
          Rs(i) = p;
          i=i+oneI32;
        end
        %leftC(1:len) = int32(linspace(c1-HALF_OFFSET, c2-HALF_OFFSET, len));
        %y = linspace(d1, d2, n)
        %y = [d1+(0:n-2)*(d2-d1)/(floor(n)-1) d2];
        
        quotient = (single(c2-c1))/(single(len)-single(1) + single(eps));%(d2-d1)/(floor(n)-1)
        for i=oneI32:len
            leftC(i)  = (c1-HALF_OFFSET) + int32((single(i)-single(1))*quotient);
            rightC(i) = leftC(i)+ twoI32*HALF_OFFSET;
            if leftC(i) < oneI32
                leftC(i) = oneI32;
                if rightC(i) < oneI32
                   rightC(i) = oneI32;
                end
            end
            if rightC(i) > cW
                rightC(i) = cW;
            end
        end
            
        whiteCount  = zeroI32;
        yellowCount = zeroI32;
        grayCount   = zeroI32;

        SumOfGotAlLeastOneWhitePixelInTheRow  = zeroI32;
        SumOfGotAlLeastOneYellowPixelInTheRow = zeroI32;
            
        for i=oneI32:len
            gotAlLeastOneWhitePixelInTheRow  = logical(false);
            gotAlLeastOneYellowPixelInTheRow = logical(false);
            for cv = leftC(i):rightC(i)
              
                   if tmpInImage_Y(Rs(i), cv) >= single(175/255)
                       whiteCount = whiteCount+oneI32;
                       gotAlLeastOneWhitePixelInTheRow = logical(true);
                   elseif tmpInImage_Cb(Rs(i), cv) >= single(90/255) && tmpInImage_Cb(Rs(i), cv) <= single(127/255) 
                       yellowCount = yellowCount+oneI32;
                       gotAlLeastOneYellowPixelInTheRow = logical(true);
                   else
                       grayCount = grayCount+oneI32;
                   end
            end
            if gotAlLeastOneWhitePixelInTheRow
              SumOfGotAlLeastOneWhitePixelInTheRow = SumOfGotAlLeastOneWhitePixelInTheRow+oneI32;
            end
            if gotAlLeastOneYellowPixelInTheRow
              SumOfGotAlLeastOneYellowPixelInTheRow = SumOfGotAlLeastOneYellowPixelInTheRow+oneI32;
            end
        end

        yellowVsTotal = single(yellowCount)/single(grayCount+yellowCount+whiteCount);
        whiteVsTotal  = single(whiteCount)/single(grayCount+yellowCount+whiteCount);
         
        if yellowVsTotal > whiteVsTotal
            lineColorIdx(lineIdx) = YELLOW_COLOR;
            linearPixelRatio = single(SumOfGotAlLeastOneYellowPixelInTheRow)/single(len);             
        else
            lineColorIdx(lineIdx) = WHITE_COLOR;
            linearPixelRatio = single(SumOfGotAlLeastOneWhitePixelInTheRow)/single(len);
        end
        
        %% distinguish solid and broken lane markers
        % if we use yellowVsTotal(==whiteVsTotal) to find marker type (solid/broken)
        % it would not give accurate result; because in the patch we are searching 
        % for yellow/white pixel- we do not know what's the pecentage of gray pixels 
        % are there
        % that's why we are considering a different method; here we try to find one
        % yellow (==white) pixel in one row; once we find a yellow (==white) pixel
        % in the row we don't need to find anything in that row of the patch (ROI)

        if linearPixelRatio > single(0.8)
             solidBrokenIdx(lineIdx) = SOLID_MARKING;
        else
             solidBrokenIdx(lineIdx) = BROKEN_MARKING;
        end 
        
        if (lineColorIdx(lineIdx) == YELLOW_COLOR) && (solidBrokenIdx(lineIdx) == BROKEN_MARKING)
            colorAndTypeIdx(lineIdx) = YELLOW_BROKEN;
        elseif (lineColorIdx(lineIdx) == YELLOW_COLOR) && (solidBrokenIdx(lineIdx) == SOLID_MARKING)
            colorAndTypeIdx(lineIdx) = YELLOW_SOLID;
        elseif (lineColorIdx(lineIdx) == WHITE_COLOR) && (solidBrokenIdx(lineIdx) == BROKEN_MARKING)
            colorAndTypeIdx(lineIdx) = WHITE_BROKEN;
        elseif (lineColorIdx(lineIdx) == WHITE_COLOR) && (solidBrokenIdx(lineIdx) == SOLID_MARKING)
            colorAndTypeIdx(lineIdx) = WHITE_SOLID;
        end
        
    else
        lineColorIdx(lineIdx) = INVALID_COLOR;
        solidBrokenIdx(lineIdx) = INVALID_MARKING;
        colorAndTypeIdx(lineIdx) = INVALID_COLOR_OR_TYPE;
    end
end
